simulink model "DC_motor_cascade"  (R2015b)
settings: Solver=VariableStepAuto  StartTime=0.0  StopTime=10  MaxStep=1e-2  RelTol=1e-3
undefined symbols (not defined in the file): P_C
settings Model: Creator=mgreiff  LastModifiedBy=mgreiff
settings DebuggingCC: AlgebraicLoopMsg=none

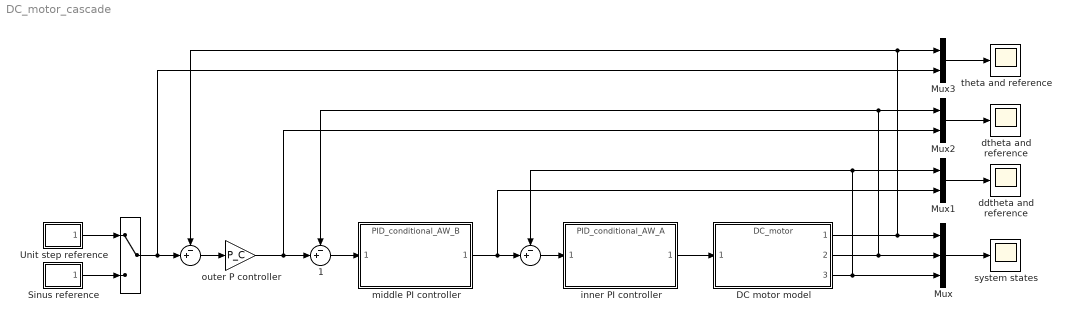
== system DC_motor_cascade ==
  " " : Sum  Inputs=-+|
  "   " : ManualSwitch
  "     " : Sum  Inputs=-+|
  " 1" : Sum  Inputs=-+|
  DC motor model : ModelReference  ModelNameDialog=DC_motor.slx  SimulationMode=Normal  ModelReferenceVersion=1.2  CopyOfModelName=DC_motor.slx
  Mux : Mux  Inputs=3
  Mux1 : Mux  Inputs=2
  Mux2 : Mux  Inputs=2
  Mux3 : Mux  Inputs=2
  Sinus reference : Subsystem
  Unit step reference : Subsystem
  ddtheta and reference : Scope
  dtheta and reference : Scope
  inner PI controller : ModelReference  ModelNameDialog=PID_conditional_AW_A.slx  SimulationMode=Normal  ModelReferenceVersion=1.2  CopyOfModelName=PID_conditional_AW_A.slx
  middle PI controller : ModelReference  ModelNameDialog=PID_conditional_AW_B.slx  SimulationMode=Normal  ModelReferenceVersion=1.2  CopyOfModelName=PID_conditional_AW_B.slx
  outer P controller : Gain  Gain=P_C
  system states : Scope
  theta and reference : Scope
  wires:
  DC motor model/1 -> Mux/1, "     "/1, Mux3/1
  DC motor model/3 -> " "/1, Mux1/1, Mux/3
  Mux/1 -> system states/1
  Unit step reference/1(voltage) -> "   "/1
  Sinus reference/1(voltage) -> "   "/2
  inner PI controller/1 -> DC motor model/1
  " "/1 -> inner PI controller/1
  Mux1/1 -> ddtheta and reference/1
  DC motor model/2 -> Mux/2, Mux2/1, " 1"/1
  Mux2/1 -> dtheta and reference/1
  middle PI controller/1 -> Mux1/2, " "/2
  " 1"/1 -> middle PI controller/1
  outer P controller/1 -> " 1"/2, Mux2/2
  "     "/1 -> outer P controller/1
  Mux3/1 -> theta and reference/1
  "   "/1 -> Mux3/2, "     "/2

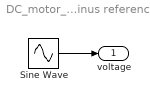
== system DC_motor_cascade/Sinus reference ==
  Sine Wave : Sin  Frequency=2*pi/10  SampleTime=0
  voltage : Outport
  wires:
  Sine Wave/1 -> voltage/1

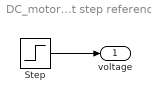
== system DC_motor_cascade/Unit step reference ==
  Step : Step  Time=0  SampleTime=0
  voltage : Outport
  wires:
  Step/1 -> voltage/1
